simulink model "OCA_SUB_modified"  (R2016a)
settings: Solver=ode3  StartTime=0.0  StopTime=100.0  RelTol=1e-3
libraries: simulink x2
settings Model: Creator=cteubert  LastModifiedBy=bourbouh
settings DataIOCC: LimitDataPoints=on
settings HardwareCC: ProdWordSize=16
settings ModelReferenceCC: PropagateSignalLabelsOutOfModel=off
settings ConfigComp: CovModelRefEnable=Off

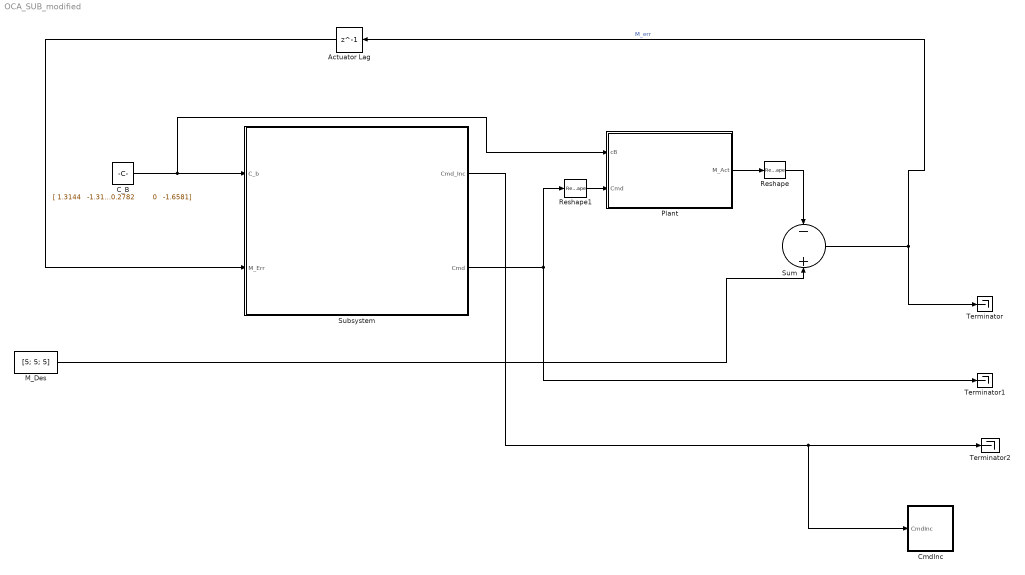
== system OCA_SUB_modified ==
  " Actuator Lag" : Delay  DelayLength=1  InitialCondition=[0;0;0]'  SampleTime=0.1
  C_B : Constant  Value=|  VectorParams1D=off
      | [ 1.3144   -1.3144         0    0.5155
      | ;         0         0   -3.9998         0;
      |     0.2782   -0.2782         0   -1.6581]
  CmdInc : Subsystem
  M_Des : Constant  Value=[5; 5; 5]
  Plant : Subsystem
  Reshape : Reshape
  Reshape1 : Reshape  OutputDimensionality=Customize  OutputDimensions=[4,1]
  Subsystem : Subsystem
  Sum : Sum  Inputs=-+
  Terminator : Terminator
  Terminator1 : Terminator
  Terminator2 : Terminator
  wires:
  Subsystem/2(Cmd) -> Reshape1/1, Terminator1/1
  Sum/1 -> " Actuator Lag"/1, Terminator/1  "M_err"
  C_B/1 -> Plant/1(cB), Subsystem/1(C_b)
  " Actuator Lag"/1 -> Subsystem/2(M_Err)
  M_Des/1 -> Sum/2
  Plant/1(M_Act) -> Reshape/1
  Reshape1/1 -> Plant/2(Cmd)
  Reshape/1 -> Sum/1
  Subsystem/1(Cmd_Inc) -> CmdInc/1("CmdInc "), Terminator2/1

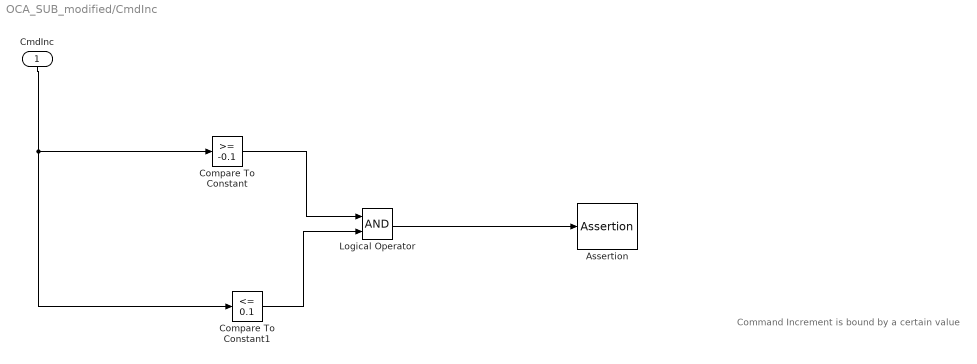
== system OCA_SUB_modified/CmdInc ==
  note: Command Increment is bound by a certain value
  "CmdInc " : Inport
  Assertion : Assertion
  Compare To Constant : simulink/Logic and Bit Operations/Compare To Constant  relop=>=  const=-0.1  OutDataTypeStr=boolean
  Compare To Constant1 : simulink/Logic and Bit Operations/Compare To Constant  relop=<=  const=0.1  OutDataTypeStr=boolean
  Logical Operator : Logic  AllPortsSameDT=off  OutDataTypeStr=boolean
  wires:
  "CmdInc "/1 -> Compare To Constant1/1, Compare To Constant/1
  Compare To Constant/1 -> Logical Operator/1
  Compare To Constant1/1 -> Logical Operator/2
  Logical Operator/1 -> Assertion/1

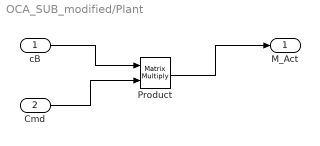
== system OCA_SUB_modified/Plant ==
  cB : Inport
  Cmd : Inport  Port=2
  Product : Product  Multiplication=Matrix(*)
  M_Act : Outport
  wires:
  Cmd/1 -> Product/2
  cB/1 -> Product/1
  Product/1 -> M_Act/1

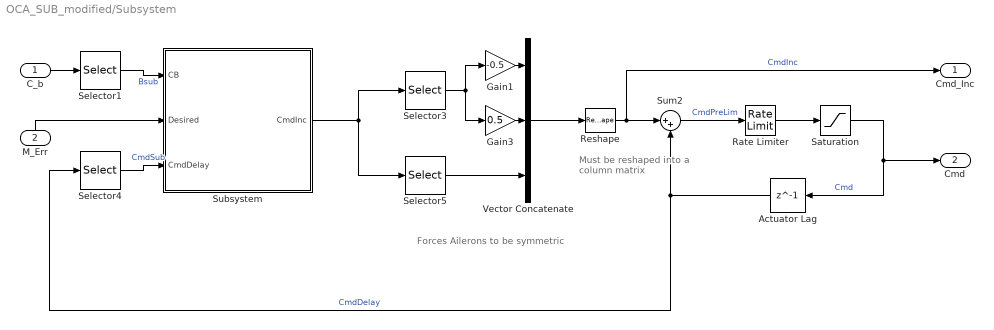
== system OCA_SUB_modified/Subsystem ==
  note: Must be reshaped into a column matrix
  note: Forces Ailerons to be symmetric
  C_b : Inport
  M_Err : Inport  Port=2
  " Actuator Lag" : Delay  DelayLength=1  InitialCondition=[0 0 0 0]'
  Gain1 : Gain  Gain=-0.5
  Gain3 : Gain  Gain=0.5
  Rate Limiter : RateLimiter  RisingSlewLimit=0.1  FallingSlewLimit=-0.1  SampleTimeMode=inherited
  Reshape : Reshape  OutputDimensionality=Column vector (2-D)
  Saturation : Saturate  UpperLimit=30  LowerLimit=-30
  Selector1 : Selector  NumberOfDimensions=2  InputPortWidth=3  IndexOptions=Select all,Index vector (dialog)  Indices=[1 3],[2:4]  OutputSizes=1,1
  Selector3 : Selector  InputPortWidth=3  IndexOptions=Index vector (dialog)  Indices=1  OutputSizes=1
  Selector4 : Selector  InputPortWidth=4  IndexOptions=Index vector (dialog)  Indices=2:4  OutputSizes=1
  Selector5 : Selector  InputPortWidth=3  IndexOptions=Index vector (dialog)  Indices=2:3  OutputSizes=1
  Subsystem : Subsystem
  Sum2 : Sum  Inputs=|++
  Vector Concatenate : Concatenate  NumInputs=3
  Cmd_Inc : Outport
  Cmd : Outport  Port=2
  wires:
  Reshape/1 -> Cmd_Inc/1, Sum2/1  "CmdInc"
  Saturation/1 -> " Actuator Lag"/1, Cmd/1  "Cmd"
  Sum2/1 -> Rate Limiter/1  "CmdPreLim"
  C_b/1 -> Selector1/1
  " Actuator Lag"/1 -> Selector4/1, Sum2/2  "CmdDelay"
  Rate Limiter/1 -> Saturation/1
  Selector1/1 -> Subsystem/1(CB)  "Bsub"
  Selector4/1 -> Subsystem/3(CmdDelay)  "CmdSub"
  Gain1/1 -> Vector Concatenate/1
  Vector Concatenate/1 -> Reshape/1
  Gain3/1 -> Vector Concatenate/2
  Selector3/1 -> Gain3/1, Gain1/1
  Selector5/1 -> Vector Concatenate/3
  Subsystem/1(CmdInc) -> Selector5/1, Selector3/1
  M_Err/1 -> Subsystem/2(Desired)

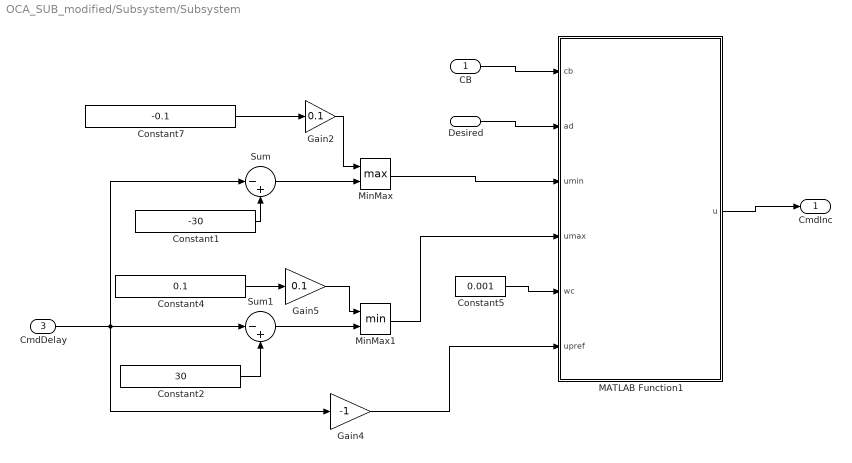
== system OCA_SUB_modified/Subsystem/Subsystem ==
  CB : Inport
  Desired : Inport  Port=2
  CmdDelay : Inport  Port=3
  Constant1 : Constant  Value=-30
  Constant2 : Constant  Value=30
  Constant4 : Constant  Value=0.1
  Constant5 : Constant  Value=0.001
  Constant7 : Constant  Value=-0.1
  Gain2 : Gain  Gain=0.1
  Gain4 : Gain  Gain=-1
  Gain5 : Gain  Gain=0.1
  MATLAB Function1 : MATLAB Function  TreatAsAtomicUnit=on
  MinMax : MinMax  Function=max  Inputs=2
  MinMax1 : MinMax  Inputs=2
  Sum : Sum  Inputs=|-+
  Sum1 : Sum  Inputs=|-+
  CmdInc : Outport
  wires:
  Constant5/1 -> MATLAB Function1/5(wc)
  MATLAB Function1/1(u) -> CmdInc/1
  Desired/1 -> MATLAB Function1/2(ad)
  CB/1 -> MATLAB Function1/1(cb)
  Gain4/1 -> MATLAB Function1/6(upref)
  Sum/1 -> MinMax/2
  Constant1/1 -> Sum/2
  Sum1/1 -> MinMax1/2
  Constant2/1 -> Sum1/2
  CmdDelay/1 -> Sum/1, Gain4/1, Sum1/1
  Constant4/1 -> Gain5/1
  Constant7/1 -> Gain2/1
  MinMax/1 -> MATLAB Function1/3(umin)
  MinMax1/1 -> MATLAB Function1/4(umax)
  Gain2/1 -> MinMax/1
  Gain5/1 -> MinMax1/1

== matlab function OCA_SUB_modified/Subsystem/Subsystem/MATLAB Function1 ==
  data: cb input; u output; ad input; umin input; umax input; wc input; upref input
function u = runOCA(cb,ad,umin,umax,wc,upref)
%#codegen

[e, u] = L1_OCA(cb,ad,umin,umax,wc,upref);
end
